simulink model "switch_led_logic"  (R2021a)
settings: Solver=FixedStepDiscrete  StartTime=0.0  StopTime=10.0  RelTol=1e-3
settings Model: Creator=U3  LastModifiedBy=U3
settings OptimizationCC: DefaultParameterBehavior=Inlined  EnhancedBackFolding=on  PassReuseOutputArgsAs=Individual arguments  ZeroExternalMemoryAtStartup=off  ZeroInternalMemoryAtStartup=off  OptimizeBlockOrder=speed  DifferentSizesBufferReuse=on  OptimizationCustomize=off  EfficientTunableParamExpr=on
settings DebuggingCC: ParameterTunabilityLossMsg=error
settings SFSimCC: MATLABDynamicMemAlloc=off
settings RTWCC: SystemTargetFile=ert.tlc  GenCodeOnly=on  TemplateMakefile=ert_default_tmf
settings CodeAppCC: ForceParamTrailComments=on  IgnoreCustomStorageClasses=off  OperatorAnnotations=on  SimulinkDataObjDesc=on  SFDataObjDesc=on  InsertBlockDesc=on
settings ERTTargetCC: TargetLangStandard=C99 (ISO)  GenerateSampleERTMain=on  InlinedParameterPlacement=NonHierarchical  ERTCustomFileTemplate=example_file_process.tlc

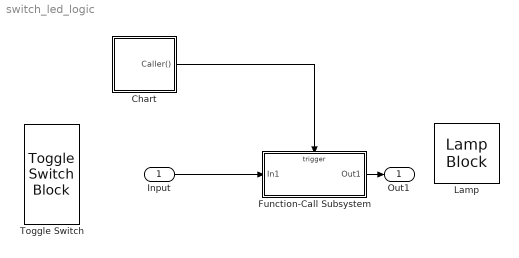
== system switch_led_logic ==
  Input : Inport
  Chart : Stateflow chart  TreatAsAtomicUnit=on
  Function-Call Subsystem : Subsystem  TreatAsAtomicUnit=on
  Lamp : LampBlock
  Toggle Switch : ToggleSwitchBlock
      settings: Values={{'Off', 'On'}, [0 1]}
  Out1 : Outport
  wires:
  Input/1 -> Function-Call Subsystem/1(In1)
  Function-Call Subsystem/1(Out1) -> Out1/1
  Chart/1(Caller()) -> Function-Call Subsystem/Trigger

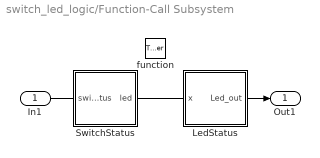
== system switch_led_logic/Function-Call Subsystem ==
  In1 : Inport
  function : TriggerPort  TriggerType=function-call  VariantControl=(inherit)
  LedStatus : Stateflow chart  TreatAsAtomicUnit=on
  SwitchStatus : Stateflow chart  TreatAsAtomicUnit=on
  Out1 : Outport
  wires:
  In1/1 -> Out1/1

== stateflow chart switch_led_logic/Chart ==
  state Counter
    en:
    du:
    ex:
  (default) -> Counter
  Counter -> Counter : [after(5,tick)]{Caller;}
  events: Caller output FUNCTION_CALL_EVENT

== stateflow chart switch_led_logic/Function-Call Subsystem/SwitchStatus ==
  note: Do not put any code along
      | the transitions that run
      | down the right side!
  (default) -> (junction 15) : /* CheckSwitch */
  (junction 15) -> (junction 16) [order 1] : [switch_status == 0]
  (junction 15) -> (junction 19) [order 2]
  (junction 16) -> (junction 17) : {led = 0;}
  (junction 17) -> (junction 18)
  (junction 18) -> (junction 22)
  (junction 19) -> (junction 20) [order 1] : [switch_status == 1]
  (junction 19) -> (junction 23) [order 2]
  (junction 20) -> (junction 21) : {led =1;}
  (junction 21) -> (junction 22)
  (junction 22) -> (junction 24)
  (junction 24) -> (junction 23)
  (junction 23) -> (junction 25)
  data: switch_status input double; led output double

== stateflow chart switch_led_logic/Function-Call Subsystem/LedStatus ==
  note: Do not put any code along
      | the transitions that run
      | down the right side!
  (default) -> (junction 40) : /* Led */
  (junction 40) -> (junction 41) [order 1] : [x == 0]
  (junction 40) -> (junction 44) [order 2]
  (junction 41) -> (junction 42) : {Led_out = 0;}
  (junction 42) -> (junction 43)
  (junction 43) -> (junction 47)
  (junction 44) -> (junction 45) [order 1] : [x == 1]
  (junction 44) -> (junction 48) [order 2]
  (junction 45) -> (junction 46) : {Led_out = 1;}
  (junction 46) -> (junction 47)
  (junction 47) -> (junction 49)
  (junction 49) -> (junction 48)
  (junction 48) -> (junction 50)
  data: x input double; Led_out output double
